simulink library "SimscapeCustomComponents_lib"  (R2025b)
settings: Solver=VariableStepAuto  StartTime=0.0  StopTime=10.0  RelTol=1e-3
undefined symbols (not defined in the file or in its folder): base, baseVdc, capacity, DiscIntNeverNeededParam, ee_sli_rtmsupport, filterInductance, freqeuncy, frequency, gcbh, gflInverter, gfmInverter, iMaxPU, Inertia, initialSOC, plantRating, solar, Ts, ups, Vac, windSystem, windTurbine
libraries: fl_lib x397, nesl_utility x171, eeGeneralControl x85, ee_lib x82, simulink x72, datacenter_lib x68, eeTransforms x38, slpidlib x24, buildingEnergy_lib x20, SimscapeFluids_lib x17, eeSinusoidalMeasurementV2 x8, eePwmGenerator x8
(part 15 of 24)

== system SimscapeCustomComponents_lib/Microgrid and Renewables/Sources/Wind Plant Integrated/Detailed/Measurements ==
  Current and Voltage Sensor (Three-Phase) : ee_lib/Sensors & Transducers/Current and Voltage Sensor (Three-Phase)  vMeasurementType=ee.enum.vmeasurement.lg  outputUnit=ee.enum.unit.pu  SRated=plantRating*1000 A*V  VRated=Vac V  I_specify=off  I_priority=None  I=[0, 0, 0] A  I_nominal_specify=off  I_nominal_value=1  I_nominal_unit=A  V_specify=off  V_priority=None  V=[0, 0, 0] V  V_nominal_specify=off  V_nominal_value=1  V_nominal_unit=V
      settings: InternalSimscapePortConfiguration="{\"Bottom\":[],\"Left\":[{\"id\":\"N1\",\"label\":\"~1\",\"type\":\"foundation.electrical.three_phase\"}],\"Right\":[{\"id\":\"V_output\",\"label\":\"V\",\"type\":\"output\"},{\"id\":\"I_output\",\"label\":\"I\",\"type\":\"output\"},{\"id\":\"N2\",\"label\":\"~2\",\"type\":\"foundation.electrical.three_phase\"}],\"Top\":[]}"
  Gain : Gain  Gain=1/(plantRating*1000)
  Gain1 : Gain  Gain=1/(plantRating*1000)
  Low-Pass Filter (Discrete or Continuous)1 : eeGeneralControl/Low-Pass Filter (Discrete or Continuous)  K=1  T=0.1  B=inf  A=-inf  init_option=Inherited from block input  x0=0  Ts=-1
  Low-Pass Filter (Discrete or Continuous)2 : eeGeneralControl/Low-Pass Filter (Discrete or Continuous)  K=1  T=0.1  B=inf  A=-inf  init_option=Inherited from block input  x0=0  Ts=-1
  PS-Simulink Converter{,1..3} (4 alike) : nesl_utility/PS-Simulink Converter  PhysicalDomain=network_engine_domain  SubClassName=ps_output  LeftPortType=input  RightPortType=output  PseudoPeriodic=off  Frequencies=[]  VectorFormat=inherit  Unit=inherit  AffineConversion=off
  Power Sensor (Three-Phase) : ee_lib/Sensors & Transducers/Power Sensor (Three-Phase)  load_type=ee.enum.passive.type_balanced.balanced  f0=60 Hz
      settings: InternalSimscapePortConfiguration="{\"Bottom\":[],\"Left\":[{\"id\":\"N1\",\"label\":\"~1\",\"type\":\"foundation.electrical.three_phase\"}],\"Right\":[{\"id\":\"N2\",\"label\":\"~2\",\"type\":\"foundation.electrical.three_phase\"}],\"Top\":[{\"id\":\"Pm\",\"label\":\"P\",\"type\":\"output\"},{\"id\":\"Qm\",\"label\":\"Q\",\"type\":\"output\"}]}"
  In : PMIOPort  Side=Left
  ~ : PMIOPort  Port=2  Side=Right
  P : Outport
  Q : Outport  Port=2
  V : Outport  Port=3
  I : Outport  Port=4
  wires:
  PS-Simulink Converter/1 -> Low-Pass Filter (Discrete or Continuous)1/1
  PS-Simulink Converter1/1 -> Low-Pass Filter (Discrete or Continuous)2/1
  Low-Pass Filter (Discrete or Continuous)1/1 -> Gain/1
  Low-Pass Filter (Discrete or Continuous)2/1 -> Gain1/1
  PS-Simulink Converter2/1 -> V/1
  PS-Simulink Converter3/1 -> I/1
  Gain/1 -> P/1
  Gain1/1 -> Q/1
  connections:
  Current and Voltage Sensor (Three-Phase)/RConn1 -- PS-Simulink Converter2/LConn1
  PS-Simulink Converter/LConn1 -- Power Sensor (Three-Phase)/LConn2
  In/RConn1 -- Power Sensor (Three-Phase)/LConn1
  Current and Voltage Sensor (Three-Phase)/RConn3 -- ~/RConn1
  PS-Simulink Converter1/LConn1 -- Power Sensor (Three-Phase)/LConn3
  Current and Voltage Sensor (Three-Phase)/LConn1 -- Power Sensor (Three-Phase)/RConn1
  Current and Voltage Sensor (Three-Phase)/RConn2 -- PS-Simulink Converter3/LConn1

== system SimscapeCustomComponents_lib/Microgrid and Renewables/Sources/Wind Plant Integrated/Detailed/PLL ==
  V : Inport
  I : Inport  Port=2
  PLL & Measurements1 : Subsystem
  VI : Outport
  wires:
  V/1 -> PLL & Measurements1/1(V)
  I/1 -> PLL & Measurements1/2(I)
  PLL & Measurements1/1(VIbus) -> VI/1

== system SimscapeCustomComponents_lib/Microgrid and Renewables/Sources/Wind Plant Integrated/Detailed/Wind Turbine and Converters ==
  note: Controller
  note: Plant
  pitch : Inport
  Wind_speed : Inport  Port=2
  LVRT : Inport  Port=3
  QRef : Inport  Port=4
  VIBus : Inport  Port=5
  Signal Conditioning : Subsystem
  Wind Controller : Subsystem  mask(Wind Controller){baseVac=Vac, baseImpedance=Vac^2/(plantRating*1000)%base.impedance, basePower=plantRating*1000, inductance=filterInductance, capacitance=0.1, Vdc=baseVoltageDC, frequency=frequency, iMaxPU=iMaxPU, mpptPower=windSystem.mpptPower, mpptWindSpeed=windSystem.mpptWindSpeed, p=p, psim=psim, Rs=Rs, Ld=Ld, Lq=Lq, airDensity=airDensity, turbineRadius=turbineRadius, pitch=pitch, TSR=TSR, cp=cp, wt=wt, rt=wt, Inertia=200, Kp_dc=0.2, Ki_dc=2, Kdpi_g=2, Kdii_g=10, Kqpi_g=2, Kqii_g=100, Kdip_sm=1, Kdii_sm=100, Kqip_sm=1, Kqii_sm=100}
      mask prompts: baseVac "Base AC Voltage (V)"; baseImpedance "Base Impedance (Ohm)"; basePower "Base Power (W)"; inductance "Filter Inductance (H)"; capacitance "DC bus capacitance (F)"; Vdc "DC bus Voltage (V)"; frequency "System Frequency (Hz)"; iMaxPU "Maximum Current (pu)"; mpptPower "MPPT Power"; mpptWindSpeed "MPPT Wind Speed"; p "Number of pole pairs"; psim "PMSM flux linkage"; Rs "Stator resistance (Ohm)"; Ld "Stator d-axis inductance (H)"; Lq "Stator q-axis inductance (H)"; airDensity "Air Density (kg/m^3)"; turbineRadius "Turbine radius (m)"; pitch "Pitch angle vector (deg)"; cp "Power Coefficient (cp)"; wt "Wind velocity threshold (m/s)"; rt "Rotational velocity threshold (rad/s)"; Inertia "Turbine Inertia (kgm^2)"; Kp_dc "Proportional gain"; Ki_dc "Integral gain"; Kdpi_g "d-axis proportional gain"; Kdii_g "d-axis integrall gain"; Kqpi_g "q-axis proportional gain"; Kqii_g "q-axis integral gain"; Kdip_sm "d-axis proportional gain"; Kdii_sm "d-axis integral gain"; Kqip_sm "q-axis proportional gain"; Kqii_sm "q-axis integral gain"
      mask help: This block implements the control strategy for a Type-4 wind turbine system, which uses a full-scale back-to-back converter to interface the generator with the grid. The controller manages both the machine-side converter (for generator torque and speed control) and the grid-side converter (for active/reactive power regulation and grid compliance). It ensures smooth power transfer, grid code adherence, and dynamic performance under varying wind and grid conditions. The design supports advanced functionalities such as fault ride-through and voltage support.
      mask DialogControl Container9 Prompt: General
      mask DialogControl Container3 Prompt: PMSM Parameters
      mask DialogControl Container4 Prompt: Wind Turbine Parameters
      mask DialogControl Container6 Prompt: Grid Side Converter Controller
      mask DialogControl Container7 Prompt: DC bus voltage controller
      mask DialogControl Container8 Prompt: Current Controller
      mask DialogControl Container10 Prompt: Machine Side Converter Controller
  Wind Plant : Subsystem  mask(Wind Plant){ratedVoltage=Vac, Vdc=baseVoltageDC, capDC=capacitance, airDensity=airDensity, turbineRadius=turbineRadius, pitch=pitch, TSR=TSR, cp=cp, wt=wt, rt=rt, p=p, psim=psim, Rs=Rs, Ld=Ld, Lq=Lq, converterFidelity=Switching, fSw=fSw}
      mask prompts: ratedVoltage "Rated voltage on AC side (V)"; Vdc "DC bus violtage (V)"; capDC "DC bus capacitance (F)"; airDensity "Air density (kg/m^3)"; turbineRadius "Turbine radius (m)"; pitch "Pitch angle vector (deg)"; TSR "Tip speed ratio"; cp "Power coefficient table, Cp(beta,TSR)"; wt "Wind velocity threshold (m/s)"; rt "Rotational velocity threshold (rad/s)"; p "Number of pole pairs"; psim "PMSM flux linkage (Wb)"; Rs "Stator resistance (Ohm)"; Ld "Stator d-axis inductance (H)"; Lq "Stator q-axis inductance (H)"; converterFidelity "Converter Fidelity"; fSw "Switching Frequency (kHz)"
      mask help: This block represents the physical interface between the wind turbine and the power converters. It models the electrical and dynamic characteristics of the wind turbine connected to a converter, while expecting an external control signal for operation
      settings: CopyFcn=set_param(gcbh,'LinkStatus','none');
      mask TypeOptions capDC: Back-to-Back Converters/capDC
      mask TypeOptions converterFidelity: Back-to-Back Converters/converterFidelity
      mask Callback converterFidelity: component.mask.setSwitchingFrequency;
      mask TypeOptions fSw: Back-to-Back Converters/fSw
      mask DialogControl Container4 Prompt: General
      mask DialogControl Container5 Prompt: Wind Turbine
      mask DialogControl editWindTurbine Prompt: Edit Wind Turbine Parameters
      mask DialogControl editWindTurbine Callback:
      | blockPath = [gcb,'/','Wind Turbine'];
      | component.mask.openBlock(blockPath);
      mask DialogControl Container6 Prompt: PMSG
      mask DialogControl editMachine Prompt: Edit PMSG Parameters
      mask DialogControl editMachine Callback:
      | blockPath = [gcb,'/','PMSG'];
      | component.mask.openBlock(blockPath);
      mask DialogControl Container7 Prompt: Converter
      mask DialogControl editMSConverter Prompt: Edit machine side converter parameters
      mask DialogControl editMSConverter Callback:
      | converterFidelity = get_param(gcb,'converterFidelity');
      | if strcmp(converterFidelity,'Average')
      |     blockPath = [gcb,'/','Back-to-Back Converters','/',converterFidelity,'/','Machine Side Converter'];
      | else
      |     blockPath = [gcb,'/','Back-to-Back Converters','/',converterFidelity,'/','Machine Side Converter','/','Converter'];
      | end
      | component.mask.openBlock(blockPath);
      mask DialogControl editGSConverter Prompt: Edit grid side converter parameters
      mask DialogControl editGSConverter Callback:
      | converterFidelity = get_param(gcb,'converterFidelity');
      | if strcmp(converterFidelity,'Average')
      |     blockPath = [gcb,'/','Back-to-Back Converters','/',converterFidelity,'/','Grid Side Converter'];
      | else
      |     blockPath = [gcb,'/','Back-to-Back Converters','/',converterFidelity,'/','Grid Side Converter','/','Converter'];
      | end
      | component.mask.openBlock(blockPath);
      mask Display: image('T4wind.png');
  ~ : PMIOPort  Side=Right
  wires:
  VIBus/1 -> Wind Controller/8(VIbus)
  QRef/1 -> Wind Controller/7(QRef)
  LVRT/1 -> Wind Controller/6(LVRT)
  Wind Controller/3(m_abc) -> Wind Plant/5(Grid)
  Wind Controller/2(SM converter control) -> Wind Plant/4(Machine)
  Wind_speed/1 -> Wind Plant/2(Wind speed)
  pitch/1 -> Wind Plant/1(Pitch)
  Wind Controller/1(Chopper Control) -> Wind Plant/3(Chopper)
  Signal Conditioning/1(iPMSM) -> Wind Controller/1(iPMSM)
  Signal Conditioning/2(rotorSpeed) -> Wind Controller/2(w)
  Signal Conditioning/3(theta) -> Wind Controller/3(theta)
  Signal Conditioning/4(Vdc) -> Wind Controller/4(vdc)
  Signal Conditioning/5(windSpeed) -> Wind Controller/5(Wind speed)
  Wind Plant/2(Meas) -> Signal Conditioning/2(Meas)
  Wind Plant/1(PMSM) -> Signal Conditioning/1(PMSM)
  connections:
  Wind Plant/RConn1 -- ~/RConn1

== system SimscapeCustomComponents_lib/Microgrid and Renewables/Sources/Wind Plant Integrated/Simplified/Measurements ==
  Current and Voltage Sensor (Three-Phase) : ee_lib/Sensors & Transducers/Current and Voltage Sensor (Three-Phase)  vMeasurementType=ee.enum.vmeasurement.lg  outputUnit=ee.enum.unit.pu  SRated=plantRating*1000 A*V  VRated=Vac V  I_specify=off  I_priority=None  I=[0, 0, 0] A  I_nominal_specify=off  I_nominal_value=1  I_nominal_unit=A  V_specify=off  V_priority=None  V=[0, 0, 0] V  V_nominal_specify=off  V_nominal_value=1  V_nominal_unit=V
      settings: InternalSimscapePortConfiguration="{\"Bottom\":[],\"Left\":[{\"id\":\"N1\",\"label\":\"~1\",\"type\":\"foundation.electrical.three_phase\"}],\"Right\":[{\"id\":\"V_output\",\"label\":\"V\",\"type\":\"output\"},{\"id\":\"I_output\",\"label\":\"I\",\"type\":\"output\"},{\"id\":\"N2\",\"label\":\"~2\",\"type\":\"foundation.electrical.three_phase\"}],\"Top\":[]}"
  Gain : Gain  Gain=1/(plantRating*1000)
  Gain1 : Gain  Gain=1/(plantRating*1000)
  Low-Pass Filter (Discrete or Continuous)1 : eeGeneralControl/Low-Pass Filter (Discrete or Continuous)  K=1  T=0.1  B=inf  A=-inf  init_option=Inherited from block input  x0=0  Ts=-1
  Low-Pass Filter (Discrete or Continuous)2 : eeGeneralControl/Low-Pass Filter (Discrete or Continuous)  K=1  T=0.1  B=inf  A=-inf  init_option=Inherited from block input  x0=0  Ts=-1
  PS-Simulink Converter{,1..3} (4 alike) : nesl_utility/PS-Simulink Converter  PhysicalDomain=network_engine_domain  SubClassName=ps_output  LeftPortType=input  RightPortType=output  PseudoPeriodic=off  Frequencies=[]  VectorFormat=inherit  Unit=inherit  AffineConversion=off
  Power Sensor (Three-Phase) : ee_lib/Sensors & Transducers/Power Sensor (Three-Phase)  load_type=ee.enum.passive.type_balanced.balanced  f0=60 Hz
      settings: InternalSimscapePortConfiguration="{\"Bottom\":[],\"Left\":[{\"id\":\"N1\",\"label\":\"~1\",\"type\":\"foundation.electrical.three_phase\"}],\"Right\":[{\"id\":\"N2\",\"label\":\"~2\",\"type\":\"foundation.electrical.three_phase\"}],\"Top\":[{\"id\":\"Pm\",\"label\":\"P\",\"type\":\"output\"},{\"id\":\"Qm\",\"label\":\"Q\",\"type\":\"output\"}]}"
  In : PMIOPort  Side=Left
  ~ : PMIOPort  Port=2  Side=Right
  P : Outport
  Q : Outport  Port=2
  V : Outport  Port=3
  I : Outport  Port=4
  wires:
  PS-Simulink Converter/1 -> Low-Pass Filter (Discrete or Continuous)1/1
  PS-Simulink Converter1/1 -> Low-Pass Filter (Discrete or Continuous)2/1
  Low-Pass Filter (Discrete or Continuous)1/1 -> Gain/1
  Low-Pass Filter (Discrete or Continuous)2/1 -> Gain1/1
  PS-Simulink Converter2/1 -> V/1
  PS-Simulink Converter3/1 -> I/1
  Gain/1 -> P/1
  Gain1/1 -> Q/1
  connections:
  Current and Voltage Sensor (Three-Phase)/RConn1 -- PS-Simulink Converter2/LConn1
  PS-Simulink Converter/LConn1 -- Power Sensor (Three-Phase)/LConn2
  In/RConn1 -- Power Sensor (Three-Phase)/LConn1
  Current and Voltage Sensor (Three-Phase)/RConn3 -- ~/RConn1
  PS-Simulink Converter1/LConn1 -- Power Sensor (Three-Phase)/LConn3
  Current and Voltage Sensor (Three-Phase)/LConn1 -- Power Sensor (Three-Phase)/RConn1
  Current and Voltage Sensor (Three-Phase)/RConn2 -- PS-Simulink Converter3/LConn1

== system SimscapeCustomComponents_lib/Microgrid and Renewables/Storage/BESS GFM Simplified/Reference Generator/If Action Subsystem ==
  PRef : Inport
  P : Inport  Port=2
  QRef : Inport  Port=3
  Q : Inport  Port=4
  Action Port : ActionPort
  Add : Sum  Inputs=-+
  Add1 : Sum  Inputs=+-
  Add2 : Sum
  Add3 : Sum  Inputs=+-
  Add4 : Sum  Inputs=-+
  Constant : Constant  Value=2*pi*frequency  SampleTime=-1
  Constant2 : Constant
  Constant3 : Constant
  Gain : Gain  Gain=activeDroop
  Gain1 : Gain  Gain=reactiveDroop
  Gain4 : Gain  Gain=Vac
  Gain5 : Gain  Gain=2*pi*frequency
  Integrator with Wrapped State (Discrete or Continuous) : eeGeneralControl/Integrator with Wrapped State (Discrete or Continuous)  LabelModeActiveChoice=Discrete  WrappedStateUpperValue=2*pi  WrappedStateLowerValue=0  x0=0  Ts=-1
  Integrator with Wrapped State (Discrete or Continuous)1 : eeGeneralControl/Integrator with Wrapped State (Discrete or Continuous)  LabelModeActiveChoice=Discrete  WrappedStateUpperValue=2*pi  WrappedStateLowerValue=0  x0=0  Ts=-1
  Saturation : Saturate  UpperLimit=1.1  LowerLimit=0.9
  Scope : Scope
      settings: ActiveDisplayYMinimum=-1  ActiveDisplayYMaximum=1  DataLoggingVariableName=ScopeData2
  Scope1 : Scope
      settings: ActiveDisplayYMinimum=-1  ActiveDisplayYMaximum=1  DataLoggingVariableName=ScopeData3
  Scope2 : Scope  NumInputPorts=2
      settings: ActiveDisplayYMinimum=-1  ActiveDisplayYMaximum=1
  Scope3 : Scope  NumInputPorts=2
      settings: ActiveDisplayYMinimum=-1  ActiveDisplayYMaximum=1  DataLoggingVariableName=ScopeData2
  Vt : Outport
  Ph : Outport  Port=2
  wires:
  Q/1 -> Scope2/2, Add1/2
  P/1 -> Scope3/2, Add/2
  Integrator with Wrapped State (Discrete or Continuous)1/1 -> Add3/2
  Constant/1 -> Integrator with Wrapped State (Discrete or Continuous)1/1
  Add3/1 -> Ph/1
  PRef/1 -> Scope3/1, Add/1
  Add/1 -> Gain/1
  Saturation/1 -> Gain4/1
  QRef/1 -> Scope2/1, Add1/1
  Gain4/1 -> Vt/1
  Gain1/1 -> Add2/1
  Constant2/1 -> Add2/2
  Integrator with Wrapped State (Discrete or Continuous)/1 -> Add3/1
  Constant3/1 -> Add4/2
  Gain5/1 -> Integrator with Wrapped State (Discrete or Continuous)/1
  Add2/1 -> Saturation/1, Scope1/1
  Add1/1 -> Gain1/1
  Gain/1 -> Add4/1
  Add4/1 -> Gain5/1, Scope/1

== system SimscapeCustomComponents_lib/Microgrid and Renewables/Storage/BESS GFM Simplified/Reference Generator/If Action Subsystem1 ==
  PRef : Inport
  P : Inport  Port=2
  VRef : Inport  Port=3
  V : Inport  Port=4
  Action Port : ActionPort
  Add : Sum  Inputs=+-
  Add1 : Sum  Inputs=+-
  Add2 : Sum
  Add3 : Sum  Inputs=+-
  Add4 : Sum  Inputs=-+
  Constant2 : Constant
  Constant3 : Constant
  Constant4 : Constant  Value=0
  Gain : Gain  Gain=reactiveDroop
  Gain1 : Gain  Gain=activeDroop
  Gain4 : Gain  Gain=systemVoltage
  Gain5 : Gain  Gain=2*pi*systemFrequency
  Integrator with Wrapped State (Discrete or Continuous) : eeGeneralControl/Integrator with Wrapped State (Discrete or Continuous)  LabelModeActiveChoice=Discrete  WrappedStateUpperValue=2*pi  WrappedStateLowerValue=0  x0=0  Ts=-1
  Saturation : Saturate  UpperLimit=1.1  LowerLimit=0.9
  Vt : Outport
  Ph : Outport  Port=2
  wires:
  Saturation/1 -> Gain4/1
  Add3/1 -> Ph/1
  PRef/1 -> Add1/1
  VRef/1 -> Add/1
  P/1 -> Add1/2
  Gain4/1 -> Vt/1
  V/1 -> Add/2
  Gain1/1 -> Add2/1
  Constant2/1 -> Add2/2
  Integrator with Wrapped State (Discrete or Continuous)/1 -> Add3/1
  Constant3/1 -> Add4/2
  Gain5/1 -> Integrator with Wrapped State (Discrete or Continuous)/1
  Add2/1 -> Saturation/1
  Add1/1 -> Gain1/1
  Gain/1 -> Add4/1
  Add4/1 -> Gain5/1
  Constant4/1 -> Add3/2
  Add/1 -> Gain/1

== system SimscapeCustomComponents_lib/Microgrid and Renewables/Storage/BESS Integrated/Detailed/BESS Controller ==
  VRef : Inport
  FRef : Inport  Port=2
  PRef : Inport  Port=3
  QRef : Inport  Port=4
  Mode : Inport  Port=5
  Reset : Inport  Port=6
  VIBus : Inport  Port=7
  Grid Following : Subsystem  VariantControl=Grid Following  mask(Grid Following Controller){mp=0.0001, mv=0.02, P=Real power, MVA=plantRating*1000, frequency=freqeuncy, zbase=Vac^2/(plantRating*1000), L=filterInductance, Imax=iMaxPU, Td=gflInverter.sensorDelay, Kpic=0.1, Kiic=1, Kd=0}
      mask prompts: mp "Real power droop cofficient"; mv "Reactive power droop cofficient"; P "Priority mode"; MVA "Base Power (V*A)"; frequency "Frequency (Hz)"; zbase "Base Impedance (Ohm)"; L "Filter Inductance (H)"; Imax "Inverter current limit (pu)"; Td "Sensor time delay (s)"; Kpic "Proportional gain"; Kiic "Integral gain"; Kd "Derevative gain"
      mask help: This block implements a Grid Following control strategy where the BESS synchronizes with an existing grid voltage and frequency. Ideal for systems where the grid is strong and the BESS acts as a power source following grid conditions.
      settings: CopyFcn=set_param(gcb,'LinkStatus','none');
      mask TypeOptions P: Real power  | Reactive power
      mask DialogControl Container4 Prompt: General
      mask DialogControl Container5 Prompt: Current Controller
      mask Display: image('gridfollowing2_2_9_7_2_1_1.png');
  Grid Forming : Subsystem  VariantControl=Grid Forming  mask(Grid Forming Controller){power=plantRating*1000, girdLineVoltage=Vac, powerFreq=frequency, dcBusVoltage=baseVoltageDC, measSampleTime=1e-3, powerControl=Virtual Synchronous Machine, activePowerSampleTime=1e-3, droopSlope=gfmInverter.droopControl.freqSlopeMp*350, droopT1=gfmInverter.droopControl.T1, droopT2=gfmInverter.droopControl.T2, droopTC=gfmInverter.droopControl.lpfTimeConst, vsmPmeasFilterTC=1e-3, vsmFreqDroop=1, vsmInertiaTC=10, vsmDampingConst=1, dampingPowerMaxLimit=0.9, dampingPowerMinLimit=-0.9, freqMeasTimeConst=1e-3, freqOption=Constant Frequency Reference, voltreference=1, QVoltFilterTC=1e-3, QVoltDroop=10, currentLimit=Current Limiting, maxSatCurrentLimit=1.2, maxVICurrentLimit=gfmInverter.currentLimit.viCurrentLimit, ctLimitVirtualImp=gfmInverter.currentLimit.virImpResistanceCoeff, ctLimitXbyR=gfmInverter.currentLimit.virImpXbyR, ctLimitDelayTime=0.1, currentSatTime=gfmInverter.currentLimit.satCurrentRunTime, currentVITimeConst=gfmInverter.currentLimit.viFilterTimeConst, voltControlTs=5e-5, vdPGain=0.1, VdIGain=1, VdMaxCt=1.2, VdMinCt=0.8, VqPGain=0.1, VqIGain=1, VqMaxCt=1.2, VqMinCt=0.8, vdvqLPFTimeConst=1e-3, currentControlTs=5e-5, filterInductance=1e-3, IdPGain=0.1, IdIGain=1, IqPGain=0.1, IqIGain=1}
      mask prompts: power "Grid forming converter power (VA)"; girdLineVoltage "Grid line voltage (V)"; powerFreq "Grid frequency (Hz)"; dcBusVoltage "DC bus voltage"; measSampleTime "Measurement sample time"; powerControl "Active Power Control"; activePowerSampleTime "Sample time (s)"; droopSlope "Power droop slope (pu, Hz/W)"; droopT1 "Lead-Lag numerator time constant (s)"; droopT2 "Lead-Lag denominator time constant (s)"; droopTC "Filter cut-off time constant (s)"; vsmPmeasFilterTC "Power measurement filter time constant (s)"; vsmFreqDroop "Frequency droop (pu,  W/Hz)"; vsmInertiaTC "Inertia constant M (pu)"; vsmDampingConst "Damping constant (pu/Hz)"; dampingPowerMaxLimit "Damping power maximum limit (pu)"; dampingPowerMinLimit "Damping power minimum limit (pu)"; freqMeasTimeConst "Frequency measurement time constant (s)"; freqOption "Damping power fequency option"; voltreference "Voltage reference value (pu)"; QVoltFilterTC "Power measurement filter time constant (s)"; QVoltDroop "Voltage droop (pu, V/VAR)"; currentLimit "Current limiting method"; maxSatCurrentLimit "Maximum current saturation (pu)"; maxVICurrentLimit "Maximum virtual impedance current (pu)"; ctLimitVirtualImp "Virtual impedance coefficient (pu.Ohm/pu.A)"; ctLimitXbyR "Virtual X/R ratio"; ctLimitDelayTime "Maximum current delay time (s)"; currentSatTime "Current limiting run time (s)"; currentVITimeConst "Filter time constant (s)"; voltControlTs "Controller sample time (s)"; vdPGain "Vd proportional gain"; VdIGain "Vd integral gain"; VdMaxCt "Vd maximum current limit (A)"; VdMinCt "Vd minimum current limit (A)"; VqPGain "Vq proportional gain"; VqIGain "Vq integral gain"; VqMaxCt "Vq maximum current limit (A)"; VqMinCt "Vq minimum current limit (A)"; vdvqLPFTimeConst "Voltage measurement filter time constant (s)"; currentControlTs "Controller sample time (s)"; filterInductance "Filter inductance (H)"; IdPGain "Id proportional gain"; IdIGain "Id integral gain"; IqPGain "Iq proportional gain"; IqIGain "Iq integral gain"
      mask help: This block implements the grid forming controller with fault ride through capability. Input to the controller are active and reactive power reference in per unit and the sensed three-phase phase current in amphere and phase voltage in volts.
      mask init: same as SimscapeCustomComponents_lib/Microgrid and Renewables/Control/BESS/Grid Forming Control
      settings: CopyFcn=set_param(gcb,'LinkStatus','none');
      mask TypeOptions powerControl: Virtual Synchronous Machine | Droop Control
      mask Callback powerControl:
      | h = Simulink.Mask.get(gcb);
      | slectedActivePowerControl=get_param(gcb,'powerControl');
      | %slectedActivePowerControl = h.Parameters(find(string({h.Parameters.Name}) == 'powerControl')).Value;
      | switch slectedActivePowerControl
      |     case 'Virtual Synchronous Machine'
      |         h.Parameters(find(string({h.Parameters.Name}) == 'droopSlope')).Visible = 'off';
      |         h.Parameters(find(string({h.Parameters.Name}) == 'droopTC')).Visible = 'off';
      |         h.Parameters(find(string({h.Parameters.Name}) == 'droopT1')).Visible = 'off';
      |         h.Parameters(find(string({h.Parameters.Name}) == 'droopT2')).Visible = 'off';
      |         h.Parameters(find(string({h.Parameters.Name}) == 'vsmPmeasFilterTC')).Visible = 'on';
      |         h.Parameters(find(string({h.Parameters.Name}) == 'vsmFreqDroop')).Visible = 'on';
      |         h.Parameters(find(string({h.Parameters.Name}) == 'vsmInertiaTC')).Visible = 'on';
      |         h.Parameters(find(string({h.Parameters.Name}) == 'vsmDampingConst')).Visible = 'on';
      |         h.Parameters(find(string({h.Parameters.Name}) == 'dampingPowerMaxLimit')).Visible = 'on';
      |         h.Parameters(find(string({h.Parameters.Name}) == 'dampingPowerMinLimit')).Visible = 'on';
      |         h.Parameters(find(string({h.Parameters.Name}) == 'freqOption')).Visible = 'on';
      |         h.Parameters(find(string({h.Parameters.Name}) == 'freqMeasTimeConst')).Visible = 'on';
      |     case 'Droop Control'
      |         h.Parameters(find(string({h.Parameters.Name}) == 'droopSlope')).Visible = 'on';
      |         h.Parameters(find(string({h.Parameters.Name}) == 'droopTC')).Visible = 'on';
      |         h.Parameters(find(string({h.Parameters.Name}) == 'droopT1')).Visible = 'on';
      |         h.Parameters(find(string({h.Parameters.Name}) == 'droopT2')).Visible = 'on';
      |         h.Parameters(find(string({h.Parameters.Name}) == 'vsmPmeasFilterTC')).Visible = 'off';
      |         h.Parameters(find(string({h.Parameters.Name}) == 'vsmFreqDroop')).Visible = 'off';
      |         h.Parameters(find(string({h.Parameters.Name}) == 'vsmInertiaTC')).Visible = 'off';
      |         h.Parameters(find(string({h.Parameters.Name}) == 'vsmDampingConst')).Visible = 'off';
      |         h.Parameters(find(string({h.Parameters.Name}) == 'dampingPowerMaxLimit')).Visible = 'off';
      |         h.Parameters(find(string({h.Parameters.Name}) == 'dampingPowerMinLimit')).Visible = 'off';
      |         h.Parameters(find(string({h.Parameters.Name}) == 'freqOption')).Visible = 'off';
      |         h.Parameters(find(string({h.Parameters.Name}) == 'freqMeasTimeConst')).Visible = 'on';
      | 
      |     otherwise
      |         disp('Choose proper active power control method')
      | end
      mask TypeOptions freqOption: Use Grid Frequency Measurement | Constant Frequency Reference
      mask TypeOptions currentLimit: Virtual Impedance | Current Limiting | Combining Virtual Impedance and Current Limiting
      mask Callback currentLimit:
      | currentLimit = 1;
      | h = Simulink.Mask.get(gcb);
      | currentLimitControl=get_param(gcb,'currentLimit');
      | %slectedActivePowerControl = h.Parameters(find(string({h.Parameters.Name}) == 'powerControl')).Value;
      | switch currentLimitControl
      |     case 'Virtual Impedance'
      |         h.Parameters(find(string({h.Parameters.Name}) == 'maxVICurrentLimit')).Visible = 'on';
      |         h.Parameters(find(string({h.Parameters.Name}) == 'ctLimitVirtualImp')).Visible = 'on';
      |         h.Parameters(find(string({h.Parameters.Name}) == 'ctLimitXbyR')).Visible = 'on';
      |         h.Parameters(find(string({h.Parameters.Name}) == 'maxSatCurrentLimit')).Visible = 'off';
      |         h.Parameters(find(string({h.Parameters.Name}) == 'ctLimitDelayTime')).Visible = 'off';
      |         h.Parameters(find(string({h.Parameters.Name}) == 'currentSatTime')).Visible = 'off';
      |         h.Parameters(find(string({h.Parameters.Name}) == 'currentVITimeConst')).Visible = 'on';
      | 
      | 
      |     case 'Current Limiting'
      |         h.Parameters(find(string({h.Parameters.Name}) == 'maxVICurrentLimit')).Visible = 'off';
      |         h.Parameters(find(string({h.Parameters.Name}) == 'ctLimitVirtualImp')).Visible = 'off';
      |         h.Parameters(find(string({h.Parameters.Name}) == 'ctLimitXbyR')).Visible = 'off';
      |         h.Parameters(find(string({h.Parameters.Name}) == 'maxSatCurrentLimit')).Visible = 'on';
      |         h.Parameters(find(string({h.Parameters.Name}) == 'ctLimitDelayTime')).Visible = 'on';
      |         h.Parameters(find(string({h.Parameters.Name}) == 'currentSatTime')).Visible = 'off';
      |         h.Parameters(find(string({h.Parameters.Name}) == 'currentVITimeConst')).Visible = 'off';
      | 
      |     case 'Combining Virtual Impedance and Current Limiting'
      |         h.Parameters(find(string({h.Parameters.Name}) == 'maxVICurrentLimit')).Visible = 'on';
      |         h.Parameters(find(string({h.Parameters.Name}) == 'ctLimitVirtualImp')).Visible = 'on';
      |         h.Parameters(find(string({h.Parameters.Name}) == 'ctLimitXbyR')).Visible = 'on';
      |         h.Parameters(find(string({h.Parameters.Name}) == 'maxSatCurrentLimit')).Visible = 'on';
      |         h.Parameters(find(string({h.Parameters.Name}) == 'ctLimitDelayTime')).Visible = 'off';
      |         h.Parameters(find(string({h.Parameters.Name}) == 'currentSatTime')).Visible = 'on';
      |         h.Parameters(find(string({h.Parameters.Name}) == 'currentVITimeConst')).Visible = 'on';
      | 
      |     otherwise
      |         disp('Choose proper current limiting method')
      | end
      mask DialogControl ParameterGroupVar Prompt: Grid Forming Control Parameters
      mask DialogControl Container8 Prompt: Grid-forming Converter Specification
      mask DialogControl Pcontrolgrp Prompt: Active Power Controller Parameters
      mask DialogControl QcontrolGrp Prompt: Reactive Power Controller Parameters
      mask DialogControl faultRideThroughGrp Prompt: Fault Ride Through Parameters
      mask DialogControl voltControlgrp Prompt: Voltage Controller Parameters
      mask DialogControl Container15currentContGrp Prompt: Current Controller Parameters
      mask Display: image('gfmGridFormingConverterVSM1_1_7_7_2_1.png');
  mabc : Outport

== system SimscapeCustomComponents_lib/Microgrid and Renewables/Storage/BESS Integrated/Detailed/BESS Plant ==
  mabc : Inport
  Battery : batteryecm_lib/Battery  Vnom=bessVoltage V  prm_dir=simscape.enum.battery.prm_dir.disabled  R1_dis=2 Ohm  R1_ch=2 Ohm  R1=0.001 Ohm  prm_AH=simscape.enum.battery.prm_AH.infinite  AH=50 A*hr  V1=11.5 V  AH1=25 A*hr  prm_R2=simscape.enum.battery.prm_R2.disabled  R2=2000 Ohm  Tmeas=298.15 K  charge_measurement_port=simscape.enum.battery.enable.yes  prm_dyn=simscape.enum.battery.prm_dyn.off  Rp1=0.005 Ohm  tau1=30 s  Rp2=0.005 Ohm  tau2=30 s  Rp3=0.005 Ohm  tau3=30 s  Rp4=0.005 Ohm  tau4=30 s  Rp5=0.005 Ohm  tau5=30 s  prm_fade=simscape.enum.battery.prm_fade.disabled  N_fade=100  AH_fade=45 A*hr  R1_fade=2.02 Ohm  R1_ch_fade=2.02 Ohm  V1_fade=10.35 V  prm_age=simscape.enum.battery.prm_age.disabled  prm_age_OCV=simscape.enum.battery.prm_age_OCV.OCV  OCV_age=0.9  SOC_age=60  Tmeas_age=298.15 K  delta_time_age_vec=[0] d  temperature_age_vec=[273] K  OCV_scaling_age=2.2134e6  OCV_offset_age=1.632e6  temp_exp_age=0.515833569 V  t_exp_age=0.75  Vnom_T2=12 V  R1_T2=2.2 Ohm  R1_T2_dis=2.2 Ohm  R1_T2_ch=2.2 Ohm  V1_T2=11.4 V  R2_T2=2200 Ohm  Rp1_T2=0.005 Ohm  tau1_T2=30 s  Rp2_T2=0.005 Ohm  tau2_T2=30 s  Rp3_T2=0.005 Ohm  tau3_T2=30 s  Rp4_T2=0.005 Ohm  tau4_T2=30 s  Rp5_T2=0.005 Ohm  tau5_T2=30 s  Tmeas2=273.15 K  thermal_port=simscape.enum.thermaleffects.omit  thermal_mass=30000 J/K  i_specify=off  i_priority=None  i=0 A  i_nominal_specify=off  i_nominal_value=1  i_nominal_unit=A  v_specify=off  v_priority=None  v=0 V  v_nominal_specify=off  v_nominal_value=1  v_nominal_unit=V  charge_specify=off  charge_priority=High  charge=50 A*hr  charge_nominal_specify=off  charge_nominal_value=1  charge_nominal_unit=A*hr  num_cycles_specify=off  num_cycles_priority=High  num_cycles=0  num_cycles_nominal_specify=off  num_cycles_nominal_value=1  num_cycles_nominal_unit=1  temperature_specify=off  temperature_priority=High  temperature=298.15 K  temperature_nominal_specify=off  temperature_nominal_value=1  temperature_nominal_unit=K
      settings: InternalSimscapePortConfiguration="{\"Bottom\":[],\"Left\":[{\"id\":\"p\",\"label\":\"+\",\"type\":\"foundation.electrical.electrical\"},{\"id\":\"q\",\"label\":\"q\",\"type\":\"output\"}],\"Right\":[{\"id\":\"n\",\"label\":\"-\",\"type\":\"foundation.electrical.electrical\"}],\"Top\":[]}"
  Converter : Subsystem  InitFcn=%solar.mask.restoreConverterLink(gcb);  Variant=on  VariantControlMode=label  LabelModeActiveChoice=Switching  mask{converterFidelity=Switching, fSw=fSw}
      mask prompts: converterFidelity "Converter Fidelity"; fSw "Switching Frequency (kHz)"
      settings: PreSaveFcn=%solar.mask.restoreConverterLink  CloseFcn=%solar.mask.restoreConverterLink
      mask TypeOptions converterFidelity: Average | Switching
      mask Callback converterFidelity: component.mask.converterFidelity(gcb);
      mask DialogControl editSwitch Prompt: Edit converter parameters
      mask DialogControl editSwitch Callback:
      | converterFidelity = get_param(gcb,'converterFidelity');
      | blockPath = [gcb,'/',converterFidelity,'/','Converter'];
      | component.mask.openBlock(blockPath);
  Electrical Reference1 : fl_lib/Electrical/Electrical Elements/Electrical Reference
  PS-Simulink Converter : nesl_utility/PS-Simulink Converter  PhysicalDomain=network_engine_domain  SubClassName=ps_output  LeftPortType=input  RightPortType=output  PseudoPeriodic=off  Frequencies=[]  VectorFormat=inherit  Unit=inherit  AffineConversion=off
  ~ : PMIOPort  Side=Right
  SOC : Outport
  wires:
  mabc/1 -> Converter/1(mabc)
  PS-Simulink Converter/1 -> SOC/1
  connections:
  Battery/RConn1 -- Electrical Reference1/LConn1 -- Converter/LConn2
  Battery/LConn1 -- Converter/LConn1
  ~/RConn1 -- Converter/RConn1
  PS-Simulink Converter/LConn1 -- Battery/LConn2

== system SimscapeCustomComponents_lib/Microgrid and Renewables/Storage/BESS Integrated/Detailed/Filter & Measurements ==
  SOC : Inport
  Current and Voltage Sensor (Three-Phase)1 : ee_lib/Sensors & Transducers/Current and Voltage Sensor (Three-Phase)  vMeasurementType=ee.enum.vmeasurement.lg  outputUnit=ee.enum.unit.pu  SRated=plantRating*1000 A*V  VRated=Vac V  I_specify=off  I_priority=None  I=[0, 0, 0] A  I_nominal_specify=off  I_nominal_value=1  I_nominal_unit=A  V_specify=off  V_priority=None  V=[0, 0, 0] V  V_nominal_specify=off  V_nominal_value=1  V_nominal_unit=V
      settings: InternalSimscapePortConfiguration="{\"Bottom\":[],\"Left\":[{\"id\":\"N1\",\"label\":\"~1\",\"type\":\"foundation.electrical.three_phase\"}],\"Right\":[{\"id\":\"V_output\",\"label\":\"V\",\"type\":\"output\"},{\"id\":\"I_output\",\"label\":\"I\",\"type\":\"output\"},{\"id\":\"N2\",\"label\":\"~2\",\"type\":\"foundation.electrical.three_phase\"}],\"Top\":[]}"
  Gain : Gain  Gain=1/(plantRating*1000)
  Gain1 : Gain  Gain=1/(plantRating*1000)
  Low-Pass Filter (Discrete or Continuous) : eeGeneralControl/Low-Pass Filter (Discrete or Continuous)  K=1  T=0.02  B=inf  A=-inf  init_option=Inherited from block input  x0=0  Ts=Ts
  Low-Pass Filter (Discrete or Continuous)1 : eeGeneralControl/Low-Pass Filter (Discrete or Continuous)  K=1  T=0.02  B=inf  A=-inf  init_option=Inherited from block input  x0=0  Ts=Ts
  PLL & Measurements : Subsystem
      mask Display: image('PLL_9_7_2.png');
  PS-Simulink Converter2 : nesl_utility_internal/PS-Simulink Converter  PhysicalDomain=network_engine_domain  SubClassName=ps_output  LeftPortType=input  RightPortType=output  PseudoPeriodic=off  Frequencies=[]  VectorFormat=1-D array  Unit=V  AffineConversion=off
  PS-Simulink Converter3 : nesl_utility_internal/PS-Simulink Converter  PhysicalDomain=network_engine_domain  SubClassName=ps_output  LeftPortType=input  RightPortType=output  PseudoPeriodic=off  Frequencies=[]  VectorFormat=1-D array  Unit=A  AffineConversion=off
  PS-Simulink Converter6 : nesl_utility_internal/PS-Simulink Converter  PhysicalDomain=network_engine_domain  SubClassName=ps_output  LeftPortType=input  RightPortType=output  PseudoPeriodic=off  Frequencies=[]  VectorFormat=1-D array  Unit=W  AffineConversion=off
  PS-Simulink Converter7 : nesl_utility_internal/PS-Simulink Converter  PhysicalDomain=network_engine_domain  SubClassName=ps_output  LeftPortType=input  RightPortType=output  PseudoPeriodic=off  Frequencies=[]  VectorFormat=1-D array  Unit=V*A  AffineConversion=off
  Power Sensor (Three-Phase)1 : ee_lib/Sensors & Transducers/Power Sensor (Three-Phase)  load_type=ee.enum.passive.type_balanced.balanced  f0=60 Hz
      settings: InternalSimscapePortConfiguration="{\"Bottom\":[],\"Left\":[{\"id\":\"N1\",\"label\":\"~1\",\"type\":\"foundation.electrical.three_phase\"}],\"Right\":[{\"id\":\"N2\",\"label\":\"~2\",\"type\":\"foundation.electrical.three_phase\"}],\"Top\":[{\"id\":\"Pm\",\"label\":\"P\",\"type\":\"output\"},{\"id\":\"Qm\",\"label\":\"Q\",\"type\":\"output\"}]}"
  RLC (Three-Phase) : ee_lib/Passive/RLC Assemblies/RLC (Three-Phase)  port_option=ee.enum.threePhasePort.composite  component_structure=ee.enum.rlc.structure.SeriesRL  R=gfmInverter.lineResistance Ohm  L=gfmInverter.L H  C=1e-6 F  R_parasitic=0 Ohm  G_parasitic=0 1/Ohm  IL_specify=on  IL_priority=None  IL=[0, 0, 0] A  IL_nominal_specify=off  IL_nominal_value=1  IL_nominal_unit=A  VC_specify=off  VC_priority=High  VC=[0, 0, 0] V  VC_nominal_specify=off  VC_nominal_value=1  VC_nominal_unit=V
      settings: InternalSimscapePortConfiguration="{\"Bottom\":[],\"Left\":[{\"id\":\"N1\",\"label\":\"~1\",\"type\":\"foundation.electrical.three_phase\"}],\"Right\":[{\"id\":\"N2\",\"label\":\"~2\",\"type\":\"foundation.electrical.three_phase\"}],\"Top\":[]}"
  In : PMIOPort  Side=Left
  ~ : PMIOPort  Port=2  Side=Right
  VIBus : Outport
  Out Bus Element : Outport  Port=2  PortName=Meas  Element=voltage
  Out Bus Element1 : Outport  Port=2  PortName=Meas  Element=current
  Out Bus Element2 : Outport  Port=2  PortName=Meas  Element=activePower
  Out Bus Element3 : Outport  Port=2  PortName=Meas  Element=reactivePower
  BusElementOut : Outport  Port=2  PortName=Meas  Element=SOC
  wires:
  PLL & Measurements/1(VIbus) -> VIBus/1
  Low-Pass Filter (Discrete or Continuous)1/1 -> Gain/1
  Low-Pass Filter (Discrete or Continuous)/1 -> Gain1/1
  PS-Simulink Converter3/1 -> PLL & Measurements/2(I), Out Bus Element1/1
  PS-Simulink Converter7/1 -> Low-Pass Filter (Discrete or Continuous)/1
  PS-Simulink Converter6/1 -> Low-Pass Filter (Discrete or Continuous)1/1
  PS-Simulink Converter2/1 -> PLL & Measurements/1(V), Out Bus Element/1
  Gain/1 -> Out Bus Element2/1
  Gain1/1 -> Out Bus Element3/1
  SOC/1 -> BusElementOut/1
  connections:
  In/RConn1 -- RLC (Three-Phase)/LConn1
  Power Sensor (Three-Phase)1/RConn1 -- ~/RConn1
  Current and Voltage Sensor (Three-Phase)1/LConn1 -- RLC (Three-Phase)/RConn1
  Power Sensor (Three-Phase)1/LConn3 -- PS-Simulink Converter7/LConn1
  Power Sensor (Three-Phase)1/LConn2 -- PS-Simulink Converter6/LConn1
  Current and Voltage Sensor (Three-Phase)1/RConn2 -- PS-Simulink Converter3/LConn1
  Current and Voltage Sensor (Three-Phase)1/RConn1 -- PS-Simulink Converter2/LConn1
  Current and Voltage Sensor (Three-Phase)1/RConn3 -- Power Sensor (Three-Phase)1/LConn1

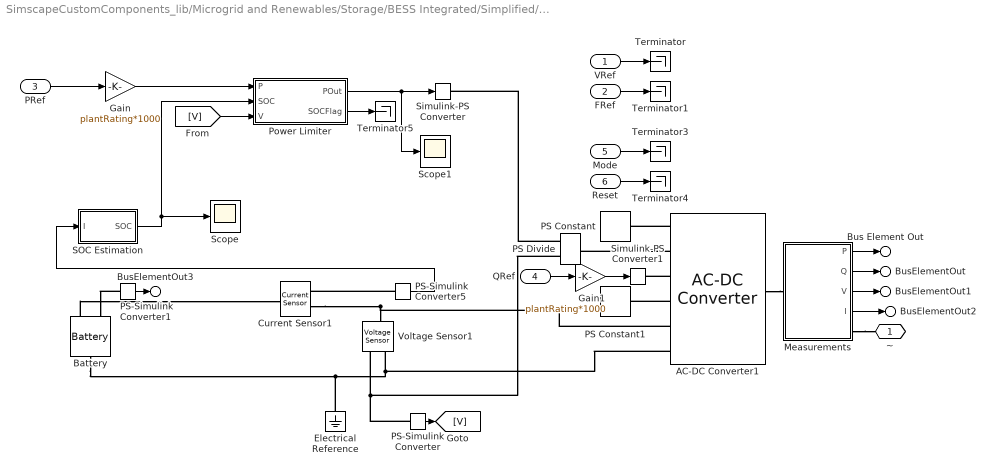
== system SimscapeCustomComponents_lib/Microgrid and Renewables/Storage/BESS Integrated/Simplified/Grid Following ==
  VRef : Inport
  FRef : Inport  Port=2
  PRef : Inport  Port=3
  QRef : Inport  Port=4
  Mode : Inport  Port=5
  Reset : Inport  Port=6
  AC-DC Converter1 : microgridRenewables_lib/AC-DC Converter  port_option=ee.enum.threePhasePort.composite  FRated=frequency Hz  Vline_rms_ini=Vac/4 V  VRated=Vac V  Vang_ini=0 deg  IMaxPU=iMaxPU  PRated=plantRating kW  efficiency=efficiency
      settings: InternalSimscapePortConfiguration="{\"Bottom\":[],\"Left\":[{\"id\":\"Vref\",\"label\":\"Vref\",\"type\":\"input\"},{\"id\":\"Iref\",\"label\":\"Iref\",\"type\":\"input\"},{\"id\":\"Qref\",\"label\":\"Qref\",\"type\":\"input\"},{\"id\":\"Mode\",\"label\":\"Mode\",\"type\":\"input\"},{\"id\":\"p\",\"label\":\"+\",\"type\":\"foundation.electrical.electrical\"},{\"id\":\"n\",\"label\":\"-\",\"type\":\"foundation.electrical.electrical\"}],\"Right\":[{\"id\":\"N\",\"label\":\"~\",\"type\":\"foundation.electrical.three_phase\"}],\"Top\":[]}"
  Battery : batteryecm_lib/Battery  Vnom=bessVoltage V  prm_dir=simscape.enum.battery.prm_dir.disabled  R1_dis=2 Ohm  R1_ch=2 Ohm  R1=1e-3 Ohm  prm_AH=simscape.enum.battery.prm_AH.infinite  AH=50 A*hr  V1=11.5 V  AH1=25 A*hr  prm_R2=simscape.enum.battery.prm_R2.disabled  R2=2000 Ohm  Tmeas=298.15 K  charge_measurement_port=simscape.enum.battery.enable.yes  prm_dyn=simscape.enum.battery.prm_dyn.off  Rp1=0.005 Ohm  tau1=30 s  Rp2=0.005 Ohm  tau2=30 s  Rp3=0.005 Ohm  tau3=30 s  Rp4=0.005 Ohm  tau4=30 s  Rp5=0.005 Ohm  tau5=30 s  prm_fade=simscape.enum.battery.prm_fade.disabled  N_fade=100  AH_fade=45 A*hr  R1_fade=2.02 Ohm  R1_ch_fade=2.02 Ohm  V1_fade=10.35 V  prm_age=simscape.enum.battery.prm_age.disabled  prm_age_OCV=simscape.enum.battery.prm_age_OCV.OCV  OCV_age=0.9  SOC_age=60  Tmeas_age=298.15 K  delta_time_age_vec=[0] d  temperature_age_vec=[273] K  OCV_scaling_age=2.2134e6  OCV_offset_age=1.632e6  temp_exp_age=0.515833569 V  t_exp_age=0.75  Vnom_T2=12 V  R1_T2=2.2 Ohm  R1_T2_dis=2.2 Ohm  R1_T2_ch=2.2 Ohm  V1_T2=11.4 V  R2_T2=2200 Ohm  Rp1_T2=0.005 Ohm  tau1_T2=30 s  Rp2_T2=0.005 Ohm  tau2_T2=30 s  Rp3_T2=0.005 Ohm  tau3_T2=30 s  Rp4_T2=0.005 Ohm  tau4_T2=30 s  Rp5_T2=0.005 Ohm  tau5_T2=30 s  Tmeas2=273.15 K  thermal_port=simscape.enum.thermaleffects.omit  thermal_mass=30000 J/K  i_specify=off  i_priority=None  i=0 A  i_nominal_specify=off  i_nominal_value=1  i_nominal_unit=A  v_specify=off  v_priority=None  v=0 V  v_nominal_specify=off  v_nominal_value=1  v_nominal_unit=V  charge_specify=off  charge_priority=High  charge=50 A*hr  charge_nominal_specify=off  charge_nominal_value=1  charge_nominal_unit=A*hr  num_cycles_specify=off  num_cycles_priority=High  num_cycles=0  num_cycles_nominal_specify=off  num_cycles_nominal_value=1  num_cycles_nominal_unit=1  temperature_specify=off  temperature_priority=High  temperature=298.15 K  temperature_nominal_specify=off  temperature_nominal_value=1  temperature_nominal_unit=K
      settings: InternalSimscapePortConfiguration="{\"Bottom\":[],\"Left\":[{\"id\":\"p\",\"label\":\"+\",\"type\":\"foundation.electrical.electrical\"},{\"id\":\"q\",\"label\":\"q\",\"type\":\"output\"}],\"Right\":[{\"id\":\"n\",\"label\":\"-\",\"type\":\"foundation.electrical.electrical\"}],\"Top\":[]}"
  Current Sensor1 : fl_lib/Electrical/Electrical Sensors/Current Sensor
  Electrical Reference : fl_lib/Electrical/Electrical Elements/Electrical Reference
  Gain : Gain  Gain=plantRating*1000
  Gain1 : Gain  Gain=plantRating*1000
  Measurements : Subsystem
  PS Constant : fl_lib/Physical Signals/Sources/PS Constant  constant=0
  PS Constant1 : fl_lib/Physical Signals/Sources/PS Constant  constant=1
  PS Divide : fl_lib/Physical Signals/Functions/PS Divide
  PS-Simulink Converter : nesl_utility/PS-Simulink Converter  PhysicalDomain=network_engine_domain  SubClassName=ps_output  LeftPortType=input  RightPortType=output  PseudoPeriodic=off  Frequencies=[]  VectorFormat=inherit  Unit=inherit  AffineConversion=off
  PS-Simulink Converter1 : nesl_utility/PS-Simulink Converter  PhysicalDomain=network_engine_domain  SubClassName=ps_output  LeftPortType=input  RightPortType=output  PseudoPeriodic=off  Frequencies=[]  VectorFormat=inherit  Unit=inherit  AffineConversion=off
  PS-Simulink Converter5 : nesl_utility/PS-Simulink Converter  PhysicalDomain=network_engine_domain  SubClassName=ps_output  LeftPortType=input  RightPortType=output  PseudoPeriodic=off  Frequencies=[]  VectorFormat=inherit  Unit=inherit  AffineConversion=off
  Power Limiter : Subsystem
  SOC Estimation : Subsystem
  Scope : Scope
      settings: ActiveDisplayYMinimum=-1  ActiveDisplayYMaximum=1  DataLoggingVariableName=ScopeData21
  Scope1 : Scope
  Simulink-PS Converter : nesl_utility/Simulink-PS Converter  PhysicalDomain=network_engine_domain  SubClassName=ps_input  LeftPortType=input  RightPortType=output  PseudoPeriodic=off  Frequencies=[]  NoiseDistribution=none  NoiseParameters=[]  Unit=V*A  AffineConversion=off  FilteringAndDerivatives=provide  SimscapeFilterOrder=1  InputFilterTimeConstant=0.001  UdotUserProvided=0
  Simulink-PS Converter1 : nesl_utility/Simulink-PS Converter  PhysicalDomain=network_engine_domain  SubClassName=ps_input  LeftPortType=input  RightPortType=output  PseudoPeriodic=off  Frequencies=[]  NoiseDistribution=none  NoiseParameters=[]  Unit=1  AffineConversion=off  FilteringAndDerivatives=provide  SimscapeFilterOrder=1  InputFilterTimeConstant=0.001  UdotUserProvided=0
  Terminator{,1,3..5} (5 alike) : Terminator
  Voltage Sensor1 : fl_lib/Electrical/Electrical Sensors/Voltage Sensor
  ~ : PMIOPort  Side=Right
  Bus Element Out : Outport  PortName=Meas  Element=activePower
  BusElementOut : Outport  PortName=Meas  Element=reactivePower
  BusElementOut1 : Outport  PortName=Meas  Element=voltage
  BusElementOut2 : Outport  PortName=Meas  Element=current
  BusElementOut3 : Outport  PortName=Meas  Element=SOC
  wires:
  Gain/1 -> Power Limiter/1(P)
  PS-Simulink Converter/1 -> [V]
  VRef/1 -> Terminator/1
  FRef/1 -> Terminator1/1
  QRef/1 -> Gain1/1
  PS-Simulink Converter5/1 -> SOC Estimation/1(I)
  Mode/1 -> Terminator3/1
  [V] -> Power Limiter/3(V)
  SOC Estimation/1(SOC) -> Power Limiter/2(SOC), Scope/1
  Reset/1 -> Terminator4/1
  Power Limiter/1(POut) -> Simulink-PS Converter/1, Scope1/1
  Power Limiter/2(SOCFlag) -> Terminator5/1
  PRef/1 -> Gain/1
  Gain1/1 -> Simulink-PS Converter1/1
  Measurements/1(P) -> Bus Element Out/1
  Measurements/3(V) -> BusElementOut1/1
  Measurements/2(Q) -> BusElementOut/1
  Measurements/4(I) -> BusElementOut2/1
  PS-Simulink Converter1/1 -> BusElementOut3/1
  connections:
  PS Divide/LConn2 -- PS-Simulink Converter/LConn1 -- Voltage Sensor1/RConn1
  Battery/RConn1 -- Electrical Reference/LConn1 -- AC-DC Converter1/LConn6 -- Voltage Sensor1/RConn2
  Current Sensor1/RConn2 -- AC-DC Converter1/LConn5 -- Voltage Sensor1/LConn1
  AC-DC Converter1/LConn4 -- PS Constant1/RConn1
  AC-DC Converter1/LConn2 -- PS Divide/RConn1
  PS-Simulink Converter5/LConn1 -- Current Sensor1/RConn1
  PS Divide/LConn1 -- Simulink-PS Converter/RConn1
  Battery/LConn1 -- Current Sensor1/LConn1
  AC-DC Converter1/LConn1 -- PS Constant/RConn1
  AC-DC Converter1/LConn3 -- Simulink-PS Converter1/RConn1
  AC-DC Converter1/RConn1 -- Measurements/LConn1
  Measurements/RConn1 -- ~/RConn1
  PS-Simulink Converter1/LConn1 -- Battery/LConn2
